simulink model "j125"  (R2021b)
settings: Solver=VariableStepAuto  StartTime=0.0  StopTime=70e-5  RelTol=1e-3
settings Model: Creator=zhonghuatu  LastModifiedBy=zhonghuatu

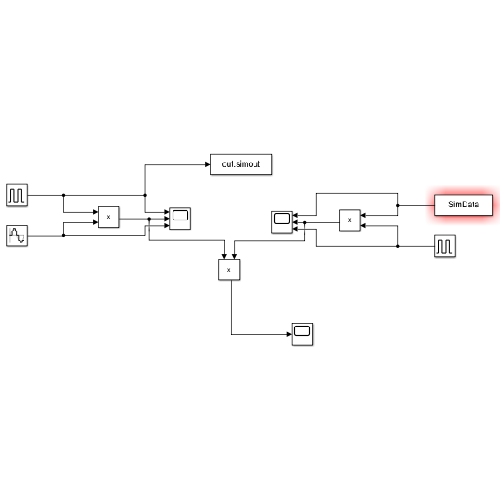
[thumbnail: Simulink's stored preview of the top-level diagram]
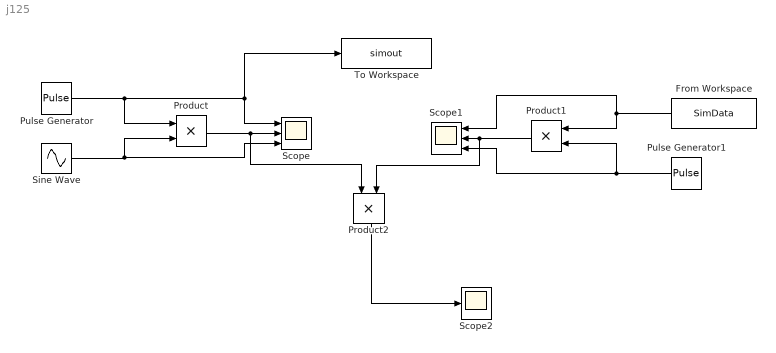
== system j125 ==
  From Workspace : FromWorkspace  VariableName=SimData
  Product : Product
  Product1 : Product
  Product2 : Product
  Pulse Generator : DiscretePulseGenerator  PulseType=Time based  Period=1e-6  PulseWidth=30
  Pulse Generator1 : DiscretePulseGenerator  PulseType=Time based  Period=1e-6  PulseWidth=30  PhaseDelay=0.2e-6
  Scope : Scope  NumInputPorts=3
  Scope1 : Scope  NumInputPorts=3
  Scope2 : Scope
  Sine Wave : Sin  Frequency=2.8e9*2*pi  SampleTime=1e-10
  To Workspace : ToWorkspace  VariableName=simout  SaveFormat=Timeseries  SampleTime=-1
  wires:
  Product/1 -> Product2/1, Scope/2
  Pulse Generator/1 -> Scope/1, To Workspace/1, Product/1
  Sine Wave/1 -> Scope/3, Product/2
  Product1/1 -> Product2/2, Scope1/2
  From Workspace/1 -> Scope1/1, Product1/1
  Pulse Generator1/1 -> Scope1/3, Product1/2
  Product2/1 -> Scope2/1
